simulink model "ModelAided_PAHRS"  (R2025b)
settings: Solver=ode4  StartTime=0.0  StopTime=300  RelTol=1e-3
values from neighbouring files (symbols this model uses):
  b_a = [0.090; -0.120; 0.075]    [Initilization.m]
  b_w = [-0.0009; 0.0010; -0.0015]    [Initilization.m]
  M_a = [50000, -15000, 10000;                   -7500, -60000, 12500;                  -12500,   5000, 20000] * 1E-6    [Initilization.m]
  M_w = [40000, -14000,  12500;                       0, -30000,  -7500;                       0,      0, -17500] * 1E-6    [Initilization.m]
libraries: slpidlib x16, simulink_extras x13, simulink x8, aerolibobsolete x4
(part 3 of 3)

== system ModelAided_PAHRS/PAHRS/Dynamic Model/Controller/theta Controller ==
  theta : Inport
  thetad : Inport  Port=2
  PID Controller : slpidlib/PID Controller  Controller=PID  Form=Parallel  TimeDomain=Continuous-time  UseExternalTs=off  SampleTime=-1  IntegratorMethod=Forward Euler  FilterMethod=Forward Euler  ControllerParametersSource=internal  P=0.000231128804122315  I=5.1930086045022e-06  UseKiTs=off  D=0.00252195493730209  UseExternalDerivativeSource=off  N=5.50508099281929  UseFilter=on  TunerSelectOption=Transfer Function Based (PID Tuner App)  InitialConditionSource=internal  InitialConditionForIntegrator=0  InitialConditionForFilter=0  DifferentiatorICPrevScaledInput=0  ExternalReset=none  TrackingMode=off  Kt=1  LimitOutput=off  SatLimitsSource=internal  UpperSaturationLimit=inf  LowerSaturationLimit=-inf  LinearizeAsGain=on  AntiWindupMode=none  Kb=1  LimitIntegrator=off  UpperIntegratorSaturationLimit=inf  LowerIntegratorSaturationLimit=-inf  POutMin=[]  POutMax=[]  IOutMin=[]  IOutMax=[]  DOutMin=[]  DOutMax=[]  NOutMin=[]  NOutMax=[]  SumOutMin=[]  SumOutMax=[]  SaturationOutMin=[]  SaturationOutMax=[]  PParamMin=[]  PParamMax=[]  IParamMin=[]  IParamMax=[]  DParamMin=[]  DParamMax=[]  NParamMin=[]  NParamMax=[]  KbParamMin=[]  KbParamMax=[]  KtParamMin=[]  KtParamMax=[]  KbOutMin=[]  KbOutMax=[]  KtOutMin=[]  KtOutMax=[]  IntegratorOutMin=[]  IntegratorOutMax=[]  FilterOutMin=[]  FilterOutMax=[]  SumI1OutMin=[]  SumI1OutMax=[]  SumI2OutMin=[]  SumI2OutMax=[]  SumI3OutMin=[]  SumI3OutMax=[]  SumI4OutMin=[]  SumI4OutMax=[]  SumDOutMin=[]  SumDOutMax=[]  DifferentiatorOutMin=[]  DifferentiatorOutMax=[]  FilterDiffOutCoefMin=[]  FilterDiffOutCoefMax=[]  ReciprocalOutMin=[]  ReciprocalOutMax=[]  SumDenOutMin=[]  SumDenOutMax=[]  SumNumOutMin=[]  SumNumOutMax=[]  DivideOutMin=[]  DivideOutMax=[]  UdiffTsProdOutMin=[]  UdiffTsProdOutMax=[]  NTsProdOutMin=[]  NTsProdOutMax=[]  UintegralTsProdOutMin=[]  UintegralTsProdOutMax=[]  UngainTsProdOutMin=[]  UngainTsProdOutMax=[]  ClampingZeroOutDataTypeStr=Inherit: Inherit via back propagation  ClampingZeroOutMin=[]  ClampingZeroOutMax=[]  FilterDenConstantOutDataTypeStr=Inherit: Inherit via back propagation  FilterDenConstantOutMin=[]  FilterDenConstantOutMax=[]  PCopyOutDataTypeStr=Inherit: Inherit via back propagation  PCopyOutMin=[]  PCopyOutMax=[]  NCopyOutDataTypeStr=Inherit: Inherit via back propagation  NCopyOutMin=[]  NCopyOutMax=[]  IntegratorContinuousStateAttributes=''  IntegratorStateMustResolveToSignalObject=off  IntegratorRTWStateStorageClass=Auto  FilterContinuousStateAttributes=''  FilterStateMustResolveToSignalObject=off  FilterRTWStateStorageClass=Auto  ParallelPVariant=InternalParameters  IdealPVariant=Disabled  IVariant=InternalParameters  DVariant=InternalParameters  IntegratorVariant=Continuous  SatVariant=Disabled  AWVariant=Passthrough  PCopyVariant=Disabled  TRVariant=Disabled  FdbkBlocksVariant=Forward  IdealPFdbkVariant=Disabled  SatFdbkVariant=Disabled  DerivativeFilterVariant=ContFilter  NVariant=InternalParameters  NCopyVariant=Disabled  FilterICVariant=InternalICsFilter  IntegratorICVariant=InternalICs  ExternalResetVariant=Disabled  TRSumVariant=Passthrough  SumFdbkVariant=Disabled  SumVariant=Sum_PID  TsampFilterVariant=InternalTs  TsampNgainVariant=Passthrough  TsampIntegralVariant=Disabled_SignalSpec  ExternalSaturationOutDataTypeStr=Inherit: Same as second input  DerivativeSourceVariant=ErrorSignal  PreIntVariant=InternalPreInt
  Sum : Sum  Inputs=|+-
  u3 : Outport
  wires:
  Sum/1 -> PID Controller/1
  PID Controller/1 -> u3/1  "u3"
  theta/1 -> Sum/2
  thetad/1 -> Sum/1

== matlab function ModelAided_PAHRS/PAHRS/Dynamic Model/Forces and Moments ==
  data: omega1 input; forces output; omega2 input; omega3 input; omega4 input; A input; moments output; V_B input; a_B output; f_prime output
function [forces, moments, a_B, f_prime] = fcn(omega1, omega2, omega3, omega4, A, V_B)
uw = 0; vw = 0; ww = 0;
u = V_B(1); v = V_B(2); w = V_B(3);
phi = A(1); theta = A(2); psi = A(3);
ua = u - uw; va = v - vw; wa = w - ww;
g = 9.81;
m = 0.296;
rho = 1.2682;
s = 0.25;
CD = 0.32;
b = 2.98e-6;
d_cg = 0.225;
d = 1.14e-7;
fx = -m*g*sin(theta) - 0.5*rho*s*CD*sqrt(ua^2+va^2+wa^2)*ua;
fy = m*g*sin(phi)*cos(theta) - 0.5*rho*s*CD*sqrt(ua^2+va^2+wa^2)*va;
fz = m*g*cos(phi)*cos(theta) - 0.5*rho*s*CD*sqrt(ua^2+va^2+wa^2)*wa - b*(omega1^2+omega2^2+omega3^2++omega4^2);
m_x = b*d_cg*(omega4^2-omega2^2);
m_y = b*d_cg*(omega1^2-omega3^2);
m_z = d*(-omega1^2+omega2^2-omega3^2+omega4^2);
forces = [fx; fy; fz];
moments = [m_x; m_y; m_z];
a_B = 1/m*[fx;fy;fz]-g*[-sin(theta); sin(phi)*cos(theta); cos(phi)*cos(theta)];

m_prime = 0.296;
s_prime = 0.25;
CD_prime = 0.32;
b_prime = 2.98e-6;
fx_prime = -m_prime*g*sin(theta) - 0.5*rho*s_prime*CD_prime*sqrt(ua^2+va^2+wa^2)*ua;
fy_prime = m_prime*g*sin(phi)*cos(theta) - 0.5*rho*s_prime*CD_prime*sqrt(ua^2+va^2+wa^2)*va;
fz_prime = m_prime*g*cos(phi)*cos(theta) - 0.5*rho*s_prime*CD_prime*sqrt(ua^2+va^2+wa^2)*wa - b_prime*(omega1^2+omega2^2+omega3^2++omega4^2);
f_prime = [fx_prime; fy_prime; fz_prime];

== matlab function ModelAided_PAHRS/PAHRS/Dynamic Model/Command Producer ==
  data: u1 input; omega12 output; omega22 output; omega32 output; omega42 output; u2 input; u3 input; u4 input
function [omega12, omega22, omega32, omega42] = fcn(u1, u2, u3, u4)
dcg = 0.225;
b = 2.98e-6;
d = 1.14e-7;
omega12 = u1/(4*b) + u3/(2*b*dcg) - u4/(4*d);
omega22 = u1/(4*b) - u2/(2*b*dcg) + u4/(4*d);
omega32 = u1/(4*b) - u3/(2*b*dcg) - u4/(4*d);
omega42 = u1/(4*b) + u2/(2*b*dcg) + u4/(4*d);

== matlab function ModelAided_PAHRS/PAHRS/PAHRS (Euler - KF - Closed Loop)/KF2/Kalman ==
  settings: updateMethod=DISCRETE
  data: omega_B input; x_prop input; deltaxhat output; y_mes input
function deltaxhat = fcn(omega_B, x_prop, y_mes)
%% Inputs
p = omega_B(1);
q = omega_B(2);
r = omega_B(3);
phi = x_prop(1);
theta = x_prop(2);
psi = x_prop(3);
persistent P
if isempty(P)
    P = 1e0*eye(1);
end
%% Propagation phase
Ts = 1;
A = [0];
B = [cos(phi)/cos(theta)];
F = eye(1) + Ts*A;
Gamma = Ts*B;
Q = 1e0*eye(1);
deltaxhat_old = zeros(1,1);
P_prop = F*P*transpose(F) + Gamma*Q*transpose(Gamma);
%% Update phase
H = eye(1);
R = 1e4*eye(1);
K = P_prop*transpose(H)*inv(H*P_prop*transpose(H)+R);
y_prop = H*x_prop(3);
deltaz = y_mes - y_prop;
P=(eye(1)-K*H)*P_prop*transpose(eye(1)-K*H)+K*R*transpose(K);
deltaxhat = deltaxhat_old + K*deltaz;
end

== matlab function ModelAided_PAHRS/PAHRS/PAHRS (Euler - KF - Closed Loop)/Enable2 ==
  data: t input; enable output
function enable = fcn(t)

if mod(t,1) == 0
    enable = 1;
else
    enable = 0;
end

== matlab function ModelAided_PAHRS/AHRS/Dynamic Model/Forces and Moments ==
  data: omega1 input; forces output; omega2 input; omega3 input; omega4 input; A input; moments output; V_B input; a_B output; f_prime output
function [forces, moments, a_B, f_prime] = fcn(omega1, omega2, omega3, omega4, A, V_B)
uw = 0; vw = 0; ww = 0;
u = V_B(1); v = V_B(2); w = V_B(3);
phi = A(1); theta = A(2); psi = A(3);
ua = u - uw; va = v - vw; wa = w - ww;
g = 9.81;
m = 0.296;
rho = 1.2682;
s = 0.25;
CD = 0.32;
b = 2.98e-6;
d_cg = 0.225;
d = 1.14e-7;
fx = -m*g*sin(theta) - 0.5*rho*s*CD*sqrt(ua^2+va^2+wa^2)*ua;
fy = m*g*sin(phi)*cos(theta) - 0.5*rho*s*CD*sqrt(ua^2+va^2+wa^2)*va;
fz = m*g*cos(phi)*cos(theta) - 0.5*rho*s*CD*sqrt(ua^2+va^2+wa^2)*wa - b*(omega1^2+omega2^2+omega3^2++omega4^2);
m_x = b*d_cg*(omega4^2-omega2^2);
m_y = b*d_cg*(omega1^2-omega3^2);
m_z = d*(-omega1^2+omega2^2-omega3^2+omega4^2);
forces = [fx; fy; fz];
moments = [m_x; m_y; m_z];
a_B = 1/m*[fx;fy;fz]-g*[-sin(theta); sin(phi)*cos(theta); cos(phi)*cos(theta)];

m_prime = 0.296;
s_prime = 0.25;
CD_prime = 0.32;
b_prime = 2.98e-6;
fx_prime = -m_prime*g*sin(theta) - 0.5*rho*s_prime*CD_prime*sqrt(ua^2+va^2+wa^2)*ua;
fy_prime = m_prime*g*sin(phi)*cos(theta) - 0.5*rho*s_prime*CD_prime*sqrt(ua^2+va^2+wa^2)*va;
fz_prime = m_prime*g*cos(phi)*cos(theta) - 0.5*rho*s_prime*CD_prime*sqrt(ua^2+va^2+wa^2)*wa - b_prime*(omega1^2+omega2^2+omega3^2++omega4^2);
f_prime = [fx_prime; fy_prime; fz_prime];

== matlab function ModelAided_PAHRS/PAHRS/Dynamic Model/Controller/MATLAB Function ==
  data: t input; phid output; thetad output; psid output
function [phid, thetad, psid] = fcn(t)

if t < 50
    phid = deg2rad(20);
    thetad = deg2rad(0);
    psid = deg2rad(0);
elseif t < 100
    phid = deg2rad(0);
    thetad = deg2rad(0);
    psid = deg2rad(0);
elseif t < 150
    phid = deg2rad(0);
    thetad = deg2rad(20);
    psid = deg2rad(0);
elseif t < 200
    phid = deg2rad(0);
    thetad = deg2rad(0);
    psid = deg2rad(0);
elseif t < 250
    phid = deg2rad(0);
    thetad = deg2rad(0);
    psid = deg2rad(90);
else 
    phid = deg2rad(0);
    thetad = deg2rad(0);
    psid = deg2rad(0);
end

== matlab function ModelAided_PAHRS/PAHRS/Dynamic Model/Controller/h Controller/ustar ==
  data: phi input; ustar output; theta input
function ustar  = fcn(phi, theta)
g = 9.81;
m = 0.336;
ustar = m * g * cos(theta) * cos(phi);

== matlab function ModelAided_PAHRS/AHRS/Dynamic Model/Controller/MATLAB Function ==
  data: t input; phid output; thetad output; psid output
function [phid, thetad, psid] = fcn(t)

if t < 50
    phid = deg2rad(20);
    thetad = deg2rad(0);
    psid = deg2rad(0);
elseif t < 100
    phid = deg2rad(0);
    thetad = deg2rad(0);
    psid = deg2rad(0);
elseif t < 150
    phid = deg2rad(0);
    thetad = deg2rad(20);
    psid = deg2rad(0);
elseif t < 200
    phid = deg2rad(0);
    thetad = deg2rad(0);
    psid = deg2rad(0);
elseif t < 250
    phid = deg2rad(0);
    thetad = deg2rad(0);
    psid = deg2rad(90);
else 
    phid = deg2rad(0);
    thetad = deg2rad(0);
    psid = deg2rad(0);
end

== matlab function ModelAided_PAHRS/AHRS/Dynamic Model/Controller/h Controller/ustar ==
  data: phi input; ustar output; theta input
function ustar  = fcn(phi, theta)
g = 9.81;
m = 0.336;
ustar = m * g * cos(theta) * cos(phi);

== matlab function ModelAided_PAHRS/Gyroscope/Dynamic Model/Command Producer ==
  data: u1 input; omega12 output; omega22 output; omega32 output; omega42 output; u2 input; u3 input; u4 input
function [omega12, omega22, omega32, omega42] = fcn(u1, u2, u3, u4)
dcg = 0.225;
b = 2.98e-6;
d = 1.14e-7;
omega12 = u1/(4*b) + u3/(2*b*dcg) - u4/(4*d);
omega22 = u1/(4*b) - u2/(2*b*dcg) + u4/(4*d);
omega32 = u1/(4*b) - u3/(2*b*dcg) - u4/(4*d);
omega42 = u1/(4*b) + u2/(2*b*dcg) + u4/(4*d);

== matlab function ModelAided_PAHRS/Gyroscope/Dynamic Model/Controller/MATLAB Function ==
  data: t input; phid output; thetad output; psid output
function [phid, thetad, psid] = fcn(t)

if t < 50
    phid = deg2rad(20);
    thetad = deg2rad(0);
    psid = deg2rad(0);
elseif t < 100
    phid = deg2rad(0);
    thetad = deg2rad(0);
    psid = deg2rad(0);
elseif t < 150
    phid = deg2rad(0);
    thetad = deg2rad(20);
    psid = deg2rad(0);
elseif t < 200
    phid = deg2rad(0);
    thetad = deg2rad(0);
    psid = deg2rad(0);
elseif t < 250
    phid = deg2rad(0);
    thetad = deg2rad(0);
    psid = deg2rad(90);
else 
    phid = deg2rad(0);
    thetad = deg2rad(0);
    psid = deg2rad(0);
end

== matlab function ModelAided_PAHRS/Gyroscope/Dynamic Model/Controller/h Controller/ustar ==
  data: phi input; ustar output; theta input
function ustar  = fcn(phi, theta)
g = 9.81;
m = 0.336;
ustar = m * g * cos(theta) * cos(phi);

== matlab function ModelAided_PAHRS/Gyroscope/Dynamic Model/Forces and Moments ==
  data: omega1 input; forces output; omega2 input; omega3 input; omega4 input; A input; moments output; V_B input; a_B output; f_prime output
function [forces, moments, a_B, f_prime] = fcn(omega1, omega2, omega3, omega4, A, V_B)
uw = 0; vw = 0; ww = 0;
u = V_B(1); v = V_B(2); w = V_B(3);
phi = A(1); theta = A(2); psi = A(3);
ua = u - uw; va = v - vw; wa = w - ww;
g = 9.81;
m = 0.296;
rho = 1.2682;
s = 0.25;
CD = 0.32;
b = 2.98e-6;
d_cg = 0.225;
d = 1.14e-7;
fx = -m*g*sin(theta) - 0.5*rho*s*CD*sqrt(ua^2+va^2+wa^2)*ua;
fy = m*g*sin(phi)*cos(theta) - 0.5*rho*s*CD*sqrt(ua^2+va^2+wa^2)*va;
fz = m*g*cos(phi)*cos(theta) - 0.5*rho*s*CD*sqrt(ua^2+va^2+wa^2)*wa - b*(omega1^2+omega2^2+omega3^2++omega4^2);
m_x = b*d_cg*(omega4^2-omega2^2);
m_y = b*d_cg*(omega1^2-omega3^2);
m_z = d*(-omega1^2+omega2^2-omega3^2+omega4^2);
forces = [fx; fy; fz];
moments = [m_x; m_y; m_z];
a_B = 1/m*[fx;fy;fz]-g*[-sin(theta); sin(phi)*cos(theta); cos(phi)*cos(theta)];

m_prime = 0.296;
s_prime = 0.25;
CD_prime = 0.32;
b_prime = 2.98e-6;
fx_prime = -m_prime*g*sin(theta) - 0.5*rho*s_prime*CD_prime*sqrt(ua^2+va^2+wa^2)*ua;
fy_prime = m_prime*g*sin(phi)*cos(theta) - 0.5*rho*s_prime*CD_prime*sqrt(ua^2+va^2+wa^2)*va;
fz_prime = m_prime*g*cos(phi)*cos(theta) - 0.5*rho*s_prime*CD_prime*sqrt(ua^2+va^2+wa^2)*wa - b_prime*(omega1^2+omega2^2+omega3^2++omega4^2);
f_prime = [fx_prime; fy_prime; fz_prime];

== matlab function ModelAided_PAHRS/Gyroscope/Propagation/Propagation1 ==
  data: A_prop output; omega_B input; A_prev input
function A_prop    = fcn(omega_B, A_prev)
%% Inputs
phi = A_prev(1);
theta = A_prev(2);
psi = A_prev(3);
p = omega_B(1);
q = omega_B(2);
r = omega_B(3);
%% Propagation
phidot = p + q*sin(phi)*tan(theta) + r*cos(phi)*tan(theta);
thetadot = q*cos(phi) - r*sin(phi);
psidot = q*sin(phi)/cos(theta) + r*cos(phi)/cos(theta);
Adot = [phidot; thetadot; psidot];
%% Update
Ts = 0.01;
A_prop = A_prev + Ts*Adot;
end

== matlab function ModelAided_PAHRS/Gravity/Dynamic Model/Command Producer ==
  data: u1 input; omega12 output; omega22 output; omega32 output; omega42 output; u2 input; u3 input; u4 input
function [omega12, omega22, omega32, omega42] = fcn(u1, u2, u3, u4)
dcg = 0.225;
b = 2.98e-6;
d = 1.14e-7;
omega12 = u1/(4*b) + u3/(2*b*dcg) - u4/(4*d);
omega22 = u1/(4*b) - u2/(2*b*dcg) + u4/(4*d);
omega32 = u1/(4*b) - u3/(2*b*dcg) - u4/(4*d);
omega42 = u1/(4*b) + u2/(2*b*dcg) + u4/(4*d);

== matlab function ModelAided_PAHRS/Gravity/Dynamic Model/Controller/MATLAB Function ==
  data: t input; phid output; thetad output; psid output
function [phid, thetad, psid] = fcn(t)

if t < 50
    phid = deg2rad(20);
    thetad = deg2rad(0);
    psid = deg2rad(0);
elseif t < 100
    phid = deg2rad(0);
    thetad = deg2rad(0);
    psid = deg2rad(0);
elseif t < 150
    phid = deg2rad(0);
    thetad = deg2rad(20);
    psid = deg2rad(0);
elseif t < 200
    phid = deg2rad(0);
    thetad = deg2rad(0);
    psid = deg2rad(0);
elseif t < 250
    phid = deg2rad(0);
    thetad = deg2rad(0);
    psid = deg2rad(90);
else 
    phid = deg2rad(0);
    thetad = deg2rad(0);
    psid = deg2rad(0);
end

== matlab function ModelAided_PAHRS/Gravity/Dynamic Model/Controller/h Controller/ustar ==
  data: phi input; ustar output; theta input
function ustar  = fcn(phi, theta)
g = 9.81;
m = 0.336;
ustar = m * g * cos(theta) * cos(phi);

== matlab function ModelAided_PAHRS/Gravity/Dynamic Model/Forces and Moments ==
  data: omega1 input; forces output; omega2 input; omega3 input; omega4 input; A input; moments output; V_B input; a_B output; f_prime output
function [forces, moments, a_B, f_prime] = fcn(omega1, omega2, omega3, omega4, A, V_B)
uw = 0; vw = 0; ww = 0;
u = V_B(1); v = V_B(2); w = V_B(3);
phi = A(1); theta = A(2); psi = A(3);
ua = u - uw; va = v - vw; wa = w - ww;
g = 9.81;
m = 0.296;
rho = 1.2682;
s = 0.25;
CD = 0.32;
b = 2.98e-6;
d_cg = 0.225;
d = 1.14e-7;
fx = -m*g*sin(theta) - 0.5*rho*s*CD*sqrt(ua^2+va^2+wa^2)*ua;
fy = m*g*sin(phi)*cos(theta) - 0.5*rho*s*CD*sqrt(ua^2+va^2+wa^2)*va;
fz = m*g*cos(phi)*cos(theta) - 0.5*rho*s*CD*sqrt(ua^2+va^2+wa^2)*wa - b*(omega1^2+omega2^2+omega3^2++omega4^2);
m_x = b*d_cg*(omega4^2-omega2^2);
m_y = b*d_cg*(omega1^2-omega3^2);
m_z = d*(-omega1^2+omega2^2-omega3^2+omega4^2);
forces = [fx; fy; fz];
moments = [m_x; m_y; m_z];
a_B = 1/m*[fx;fy;fz]-g*[-sin(theta); sin(phi)*cos(theta); cos(phi)*cos(theta)];

m_prime = 0.296;
s_prime = 0.25;
CD_prime = 0.32;
b_prime = 2.98e-6;
fx_prime = -m_prime*g*sin(theta) - 0.5*rho*s_prime*CD_prime*sqrt(ua^2+va^2+wa^2)*ua;
fy_prime = m_prime*g*sin(phi)*cos(theta) - 0.5*rho*s_prime*CD_prime*sqrt(ua^2+va^2+wa^2)*va;
fz_prime = m_prime*g*cos(phi)*cos(theta) - 0.5*rho*s_prime*CD_prime*sqrt(ua^2+va^2+wa^2)*wa - b_prime*(omega1^2+omega2^2+omega3^2++omega4^2);
f_prime = [fx_prime; fy_prime; fz_prime];

== matlab function ModelAided_PAHRS/Gravity/PAHRS (Euler - KF - Closed Loop)/Enable1 ==
  data: t input; enable output
function enable = fcn(t)

if mod(t,0.01) == 0
    enable = 1;
else
    enable = 0;
end

== matlab function ModelAided_PAHRS/Gravity/PAHRS (Euler - KF - Closed Loop)/Enable2 ==
  data: t input; enable output
function enable = fcn(t)

if mod(t,1) == 0
    enable = 1;
else
    enable = 0;
end

== matlab function ModelAided_PAHRS/AHRS/AHRS (Euler - KF - Closed Loop)/Measurement/Measurement ==
  data: a_B input; phi_mes output; theta_mes output; f_B input; psi_mes input; psi_mes output
function [phi_mes, theta_mes, psi_mes] = fcn(a_B, f_B, psi_mes)
%% Inputs
g = 9.81;
m = 0.296;
ax=a_B(1);
ay=a_B(2);
az=a_B(3);
% mx=m_B(1);
% my=m_B(2);
% mz=m_B(3);
fx = f_B(1);
fy = f_B(2);
fz = f_B(3);
%% Measurement
theta_mes = -asin(-(ax-1/m*fx)/(g));
phi_mes = atan2(-(ay-1/m*fy),-(az-1/m*fz));
psi_mes = psi_mes;
% num_psi = -my*cos(phi_mes)+mz*sin(phi_mes);
% den_psi = mx*cos(theta_mes)+my*sin(theta_mes)*sin(phi_mes)+mz*sin(theta_mes)*cos(phi_mes);
% psi_mes = declination+atan2(num_psi,den_psi);
end

== matlab function ModelAided_PAHRS/Gravity/PAHRS (Euler - KF - Closed Loop)/KF1/Kalman ==
  settings: updateMethod=DISCRETE
  data: omega_B input; x_prop input; deltaxhat output; y_mes input
function deltaxhat = fcn(omega_B, x_prop, y_mes)
%% Inputs
p = omega_B(1);
q = omega_B(2);
r = omega_B(3);
phi = x_prop(1);
theta = x_prop(2);
psi = x_prop(3);
persistent P
if isempty(P)
    P = 1e0*eye(2);
end
%% Propagation phase
Ts = 0.01;
A = [(q*cos(phi)-r*sin(phi))*tan(theta), (r*cos(phi)+q*sin(phi))*(1+tan(theta)^2);
    (-r*cos(phi)-q*sin(phi)), 0];
B = [1, sin(phi)*tan(theta);
    0, cos(phi)];
F = eye(2) + Ts*A;
Gamma = Ts*B;
Q = 1e0*eye(2);
deltaxhat_old = zeros(2,1);
P_prop = F*P*transpose(F) + Gamma*Q*transpose(Gamma);
%% Update phase
H = eye(2);
R = 1e-2*eye(2);
K = P_prop*transpose(H)*inv(H*P_prop*transpose(H)+R);
y_prop = H*x_prop(1:2);
deltaz = y_mes - y_prop;
P=(eye(2)-K*H)*P_prop*transpose(eye(2)-K*H)+K*R*transpose(K);
deltaxhat = deltaxhat_old + K*deltaz;
end

== matlab function ModelAided_PAHRS/Gravity/PAHRS (Euler - KF - Closed Loop)/KF2/Kalman ==
  settings: updateMethod=DISCRETE
  data: omega_B input; x_prop input; deltaxhat output; y_mes input
function deltaxhat = fcn(omega_B, x_prop, y_mes)
%% Inputs
p = omega_B(1);
q = omega_B(2);
r = omega_B(3);
phi = x_prop(1);
theta = x_prop(2);
psi = x_prop(3);
persistent P
if isempty(P)
    P = 1e0*eye(1);
end
%% Propagation phase
Ts = 1;
A = [0];
B = [cos(phi)/cos(theta)];
F = eye(1) + Ts*A;
Gamma = Ts*B;
Q = 1e0*eye(1);
deltaxhat_old = zeros(1,1);
P_prop = F*P*transpose(F) + Gamma*Q*transpose(Gamma);
%% Update phase
H = eye(1);
R = 1e4*eye(1);
K = P_prop*transpose(H)*inv(H*P_prop*transpose(H)+R);
y_prop = H*x_prop(3);
deltaz = y_mes - y_prop;
P=(eye(1)-K*H)*P_prop*transpose(eye(1)-K*H)+K*R*transpose(K);
deltaxhat = deltaxhat_old + K*deltaz;
end

== matlab function ModelAided_PAHRS/Gravity/PAHRS (Euler - KF - Closed Loop)/Measurement/Measurement ==
  data: a_B input; phi_mes output; theta_mes output; f_B input
function [phi_mes, theta_mes] = fcn(a_B, f_B)
%% Inputs
g = 9.81;
m = 0.296;
ax=a_B(1);
ay=a_B(2);
az=a_B(3);
fx = f_B(1);
fy = f_B(2);
fz = f_B(3);
%% Measurement
theta_mes = -asin(-(ax)/(g));
phi_mes = atan2(-(ay),-(az));
end

== matlab function ModelAided_PAHRS/Gravity/PAHRS (Euler - KF - Closed Loop)/Propagation/Propagation ==
  data: A_prop output; omega_B input; Ahat input
function A_prop    = fcn(omega_B, Ahat)
%% Inputs
phi = Ahat(1);
theta = Ahat(2);
psi = Ahat(3);
p = omega_B(1);
q = omega_B(2);
r = omega_B(3);
%% Propagation
phidot = p + q*sin(phi)*tan(theta) + r*cos(phi)*tan(theta);
thetadot = q*cos(phi) - r*sin(phi);
psidot = q*sin(phi)/cos(theta) + r*cos(phi)/cos(theta);
Adot = [phidot; thetadot; psidot];
%% Update
Ts = 0.01;
A_prop = Ahat + Ts*Adot;
end

== matlab function ModelAided_PAHRS/PAHRS/PAHRS (Euler - KF - Closed Loop)/Measurement/psi_mes ==
  data: psi_mes1 input; y_mes2 output; psi_mes2 input; xhat input
function y_mes2 = fcn(psi_mes1, psi_mes2, xhat)

if abs(wrapToPi(psi_mes1-xhat(3))) < abs(wrapToPi(psi_mes2-xhat(3)))
    y_mes2 = psi_mes1;
else
    y_mes2 = psi_mes2;
end

== matlab function ModelAided_PAHRS/Gravity/PAHRS (Euler - KF - Closed Loop)/Measurement/psi_mes ==
  data: psi_mes1 input; y_mes2 output; psi_mes2 input; xhat input
function y_mes2 = fcn(psi_mes1, psi_mes2, xhat)

if abs(wrapToPi(psi_mes1-xhat(3))) < abs(wrapToPi(psi_mes2-xhat(3)))
    y_mes2 = psi_mes1;
else
    y_mes2 = psi_mes2;
end

== matlab function ModelAided_PAHRS/AHRS/Dynamic Model/Accelerometer ==
  data: a_true input; n_a input; a_B output; M_a input; b_a input
function a_B = fcn(a_true, n_a, M_a, b_a)

a_B = M_a * a_true + b_a + n_a;

== matlab function ModelAided_PAHRS/AHRS/Dynamic Model/Gytoscope ==
  data: w_true input; n_w input; w_B output; M_w input; b_w input
function w_B = fcn(w_true, n_w, M_w, b_w)

w_B = M_w * w_true + b_w + n_w;

== matlab function ModelAided_PAHRS/PAHRS/Dynamic Model/Accelerometer ==
  data: a_true input; n_a input; a_B output; M_a input; b_a input
function a_B = fcn(a_true, n_a, M_a, b_a)

a_B = (M_a+eye(3)) * a_true + b_a + n_a;

== matlab function ModelAided_PAHRS/PAHRS/Dynamic Model/Gytoscope ==
  data: w_true input; n_w input; w_B output; M_w input; b_w input
function w_B = fcn(w_true, n_w, M_w, b_w)

w_B = (M_w+eye(3)) * w_true + b_w + n_w;

== matlab function ModelAided_PAHRS/Gravity/Dynamic Model/Accelerometer ==
  data: a_true input; n_a input; a_B output; M_a input; b_a input
function a_B = fcn(a_true, n_a, M_a, b_a)

a_B = (M_a+eye(3)) * a_true + b_a + n_a;

== matlab function ModelAided_PAHRS/Gyroscope/Dynamic Model/Gytoscope ==
  data: w_true input; n_w input; w_B output; M_w input; b_w input
function w_B = fcn(w_true, n_w, M_w, b_w)

w_B = (M_w+eye(3)) * w_true + b_w + n_w;

== matlab function ModelAided_PAHRS/PAHRS/PAHRS (Euler - KF - Closed Loop)/Enable1 ==
  data: t input; enable output
function enable = fcn(t)

if mod(t,0.01) == 0
    enable = 1;
else
    enable = 0;
end

== matlab function ModelAided_PAHRS/Gravity/Dynamic Model/Gytoscope ==
  data: w_true input; n_w input; w_B output; M_w input; b_w input
function w_B = fcn(w_true, n_w, M_w, b_w)

w_B = (M_w+eye(3)) * w_true + b_w + n_w;

== matlab function ModelAided_PAHRS/PAHRS/PAHRS (Euler - KF - Closed Loop)/KF1/Kalman ==
  settings: updateMethod=DISCRETE
  data: omega_B input; x_prop input; deltaxhat output; y_mes input
function deltaxhat = fcn(omega_B, x_prop, y_mes)
%% Inputs
p = omega_B(1);
q = omega_B(2);
r = omega_B(3);
phi = x_prop(1);
theta = x_prop(2);
psi = x_prop(3);
persistent P
if isempty(P)
    P = 1e0*eye(2);
end
%% Propagation phase
Ts = 0.01;
A = [(q*cos(phi)-r*sin(phi))*tan(theta), (r*cos(phi)+q*sin(phi))*(1+tan(theta)^2);
    (-r*cos(phi)-q*sin(phi)), 0];
B = [1, sin(phi)*tan(theta);
    0, cos(phi)];
F = eye(2) + Ts*A;
Gamma = Ts*B;
Q = 1e0*eye(2);
deltaxhat_old = zeros(2,1);
P_prop = F*P*transpose(F) + Gamma*Q*transpose(Gamma);
%% Update phase
H = eye(2);
R = 1e-2*eye(2);
K = P_prop*transpose(H)*inv(H*P_prop*transpose(H)+R);
y_prop = H*x_prop(1:2);
deltaz = y_mes - y_prop;
P=(eye(2)-K*H)*P_prop*transpose(eye(2)-K*H)+K*R*transpose(K);
deltaxhat = deltaxhat_old + K*deltaz;
end

== matlab function ModelAided_PAHRS/AHRS/AHRS (Euler - KF - Closed Loop)/Propagation/Propagation ==
  data: A_prop output; omega_B input; Ahat input
function A_prop    = fcn(omega_B, Ahat)
%% Inputs
m = 0.296;
% u = V_Bhat(1);
% v = V_Bhat(2);
% w = V_Bhat(3);
phi = Ahat(1);
theta = Ahat(2);
psi = Ahat(3);
% fx = f_B(1);
% fy = f_B(2);
% fz = f_B(3);
p = omega_B(1);
q = omega_B(2);
r = omega_B(3);
%% Propagation
% udot = 1/m*fx + (r*v-q*w);
% vdot = 1/m*fy + (p*w-r*u);
% wdot = 1/m*fz + (q*u-p*v);
% V_Bdot = [udot; vdot; wdot];
phidot = p + q*sin(phi)*tan(theta) + r*cos(phi)*tan(theta);
thetadot = q*cos(phi) - r*sin(phi);
psidot = q*sin(phi)/cos(theta) + r*cos(phi)/cos(theta);
Adot = [phidot; thetadot; psidot];
%% Update
Ts = 0.01;
% V_B_prop = V_Bhat + Ts*V_Bdot;
A_prop = Ahat + Ts*Adot;
end

== matlab function ModelAided_PAHRS/PAHRS/PAHRS (Euler - KF - Closed Loop)/Measurement/Measurement ==
  data: a_B input; phi_mes output; theta_mes output; f_B input
function [phi_mes, theta_mes] = fcn(a_B, f_B)
%% Inputs
g = 9.81;
m = 0.296;
ax=a_B(1);
ay=a_B(2);
az=a_B(3);
fx = f_B(1);
fy = f_B(2);
fz = f_B(3);
%% Measurement
theta_mes = -asin(-(ax-1/m*fx)/(g));
phi_mes = atan2(-(ay-1/m*fy),-(az-1/m*fz));
end

== matlab function ModelAided_PAHRS/AHRS/AHRS (Euler - KF - Closed Loop)/KF/Kalman ==
  settings: updateMethod=DISCRETE
  data: omega_B input; x_prop input; deltaxhat output; y_mes input
function deltaxhat = fcn(omega_B, x_prop, y_mes)
%% Inputs
m = 0.296;
p = omega_B(1);
q = omega_B(2);
r = omega_B(3);
phi = x_prop(1);
theta = x_prop(2);
psi = x_prop(3);
persistent P
if isempty(P)
    P = 1e0*eye(3);
end
%% Propagation phase
Ts = 0.01;
A = [(q*cos(phi)-r*sin(phi))*tan(theta), (r*cos(phi)+q*sin(phi))*(1+tan(theta)^2), 0;
    (-r*cos(phi)-q*sin(phi)), 0, 0;
    (q*cos(phi)-r*sin(phi))/cos(theta), (r*cos(phi)+q*sin(phi))*tan(theta)/cos(theta), 0];
B = [1, sin(phi)*tan(theta), cos(phi)*tan(theta);
    0, cos(phi), -sin(phi);
    0, sin(phi)/cos(theta), cos(phi)/cos(theta)];
F = eye(3) + Ts*A;
Gamma = Ts*B;
Q = 1e-4*eye(3);
deltaxhat_old = zeros(3,1);
P_prop = F*P*transpose(F) + Gamma*Q*transpose(Gamma);
%% Update phase
H = [eye(3)];
R = 1e-6*eye(3);
K = P_prop*transpose(H)*inv(H*P_prop*transpose(H)+R);
y_prop = H*x_prop;
deltaz = y_mes - y_prop;
P=(eye(3)-K*H)*P_prop*transpose(eye(3)-K*H)+K*R*transpose(K);
deltaxhat = deltaxhat_old + K*deltaz;
end

== matlab function ModelAided_PAHRS/PAHRS/PAHRS (Euler - KF - Closed Loop)/Propagation/Propagation ==
  data: A_prop output; omega_B input; Ahat input
function A_prop    = fcn(omega_B, Ahat)
%% Inputs
phi = Ahat(1);
theta = Ahat(2);
psi = Ahat(3);
p = omega_B(1);
q = omega_B(2);
r = omega_B(3);
%% Propagation
phidot = p + q*sin(phi)*tan(theta) + r*cos(phi)*tan(theta);
thetadot = q*cos(phi) - r*sin(phi);
psidot = q*sin(phi)/cos(theta) + r*cos(phi)/cos(theta);
Adot = [phidot; thetadot; psidot];
%% Update
Ts = 0.01;
A_prop = Ahat + Ts*Adot;
end

== matlab function ModelAided_PAHRS/AHRS/AHRS (Euler - KF - Closed Loop)/Enable ==
  data: t input; enable output
function enable = fcn(t)

if mod(t,0.01) == 0
    enable = 1;
else
    enable = 0;
end

== matlab function ModelAided_PAHRS/AHRS/Dynamic Model/Command Producer ==
  data: u1 input; omega12 output; omega22 output; omega32 output; omega42 output; u2 input; u3 input; u4 input
function [omega12, omega22, omega32, omega42] = fcn(u1, u2, u3, u4)
dcg = 0.225;
b = 2.98e-6;
d = 1.14e-7;
omega12 = u1/(4*b) + u3/(2*b*dcg) - u4/(4*d);
omega22 = u1/(4*b) - u2/(2*b*dcg) + u4/(4*d);
omega32 = u1/(4*b) - u3/(2*b*dcg) - u4/(4*d);
omega42 = u1/(4*b) + u2/(2*b*dcg) + u4/(4*d);
